simulink model "sma_simulator"  (R2019b)
settings: Solver=VariableStepAuto  StartTime=0.0  StopTime=200  FixedStep=0.01  MaxStep=0.01  RelTol=1e-3
PreLoadFcn:
  | load bus_type
model workspace (MAT data in the model file):
  Af = Simulink.Parameter
  Af.Value = 44.55
  Af.DataType = 'auto'
  Af.Dimensions = [1 1]
  As = Simulink.Parameter
  As.Value = 40.83
  As.DataType = 'auto'
  As.Dimensions = [1 1]
  C1 = Simulink.Parameter
  C1.Value = Simulink.data.Expression
  C1.Value.ExpressionString = " 8 * W_c * D_s / (pi * d_s^3)"
  C1.DataType = 'auto'
  C1.Dimensions = -1
  C2 = Simulink.Parameter
  C2.Value = Simulink.data.Expression
  C2.Value.ExpressionString = " d_s / (pi * N * D_s^2)"
  C2.DataType = 'auto'
  C2.Dimensions = -1
  C_A = Simulink.Parameter
  C_A.Value = 39.55
  C_A.DataType = 'auto'
  C_A.Dimensions = [1 1]
  C_M = Simulink.Parameter
  C_M.Value = 11.51
  C_M.DataType = 'auto'
  C_M.Dimensions = [1 1]
  D_s = Simulink.Parameter
  D_s.Value = Simulink.data.Expression
  D_s.Value.ExpressionString = "d_s+4.75e-3"
  D_s.DataType = 'auto'
  D_s.Dimensions = -1
  G_A = Simulink.Parameter
  G_A.Value = 18750000000
  G_A.DataType = 'auto'
  G_A.Dimensions = [1 1]
  G_M = Simulink.Parameter
  G_M.Value = 14390000000
  G_M.DataType = 'auto'
  G_M.Dimensions = [1 1]
  Mf = Simulink.Parameter
  Mf.Value = 26.41
  Mf.DataType = 'auto'
  Mf.Dimensions = [1 1]
  Ms = Simulink.Parameter
  Ms.Value = 29.74
  Ms.DataType = 'auto'
  Ms.Dimensions = [1 1]
  N = Simulink.Parameter
  N.Value = 25
  N.DataType = 'auto'
  N.Dimensions = [1 1]
  R = Simulink.Parameter
  R.Value = Simulink.data.Expression
  R.Value.ExpressionString = "D_s/d_s"
  R.DataType = 'auto'
  R.Dimensions = -1
  Sig = Simulink.Signal
  Sig.DataType = 'auto'
  Sig.Dimensions = -1
  Sig.DimensionsMode = 'auto'
  Sig.Complexity = 'auto'
  Sig.SampleTime = -1
  Sig.SamplingMode = 'auto'
  W_c = Simulink.Parameter
  W_c.Value = Simulink.data.Expression
  W_c.Value.ExpressionString = "(4*R-1)/(4*R-4)+0.615/R"
  W_c.DataType = 'auto'
  W_c.Dimensions = -1
  a_A = Simulink.Parameter
  a_A.Value = Simulink.data.Expression
  a_A.Value.ExpressionString = "pi/(Af - As)"
  a_A.DataType = 'auto'
  a_A.Dimensions = -1
  a_M = Simulink.Parameter
  a_M.Value = Simulink.data.Expression
  a_M.Value.ExpressionString = "pi/(Ms - Mf)"
  a_M.DataType = 'auto'
  a_M.Dimensions = -1
  d_s = Simulink.Parameter
  d_s.Value = 0.0015
  d_s.DataType = 'auto'
  d_s.Dimensions = [1 1]
  gamma_L = Simulink.Parameter
  gamma_L.Value = 0.02
  gamma_L.DataType = 'auto'
  gamma_L.Dimensions = [1 1]
  tau_fcr = Simulink.Parameter
  tau_fcr.Value = 320000000
  tau_fcr.DataType = 'auto'
  tau_fcr.Dimensions = [1 1]
  tau_scr = Simulink.Parameter
  tau_scr.Value = 60000000
  tau_scr.DataType = 'auto'
  tau_scr.Dimensions = [1 1]
undefined symbols (not defined in the file or in its folder): sigbuilder_block
libraries: simulink x3
Description:
  | -> System Requirement <-
  | - Matlab 2019b
  | - Simulink with licence to
  |   - Stateflow
settings Model: PauseTimes=128  OrderedModelArguments=off  Creator=Quinn Ding  LastModifiedBy=Quinn

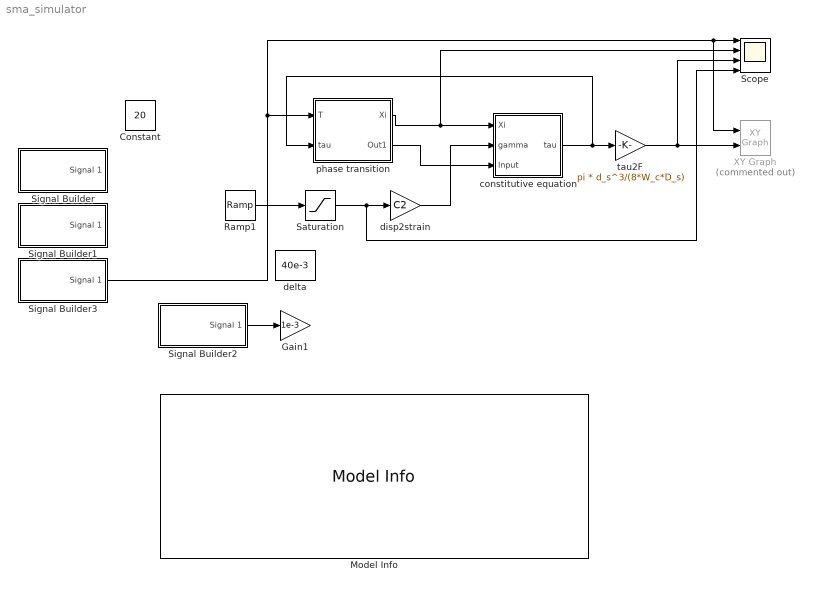
== system sma_simulator ==
  Constant : Constant  Value=20
  Gain1 : Gain  Gain=1e-3
  Model Info : simulink/Model-Wide Utilities/Model Info  Frame=on  DisplayStringWithTags=|  HorizontalTextAlignment=Left  LeftAlignmentValue=0.02
      | Shape Memory Alloy Simulator %<ModelVersion>
      | 
      | Developed by %<Creator> at Surgical Robotics & Devices Laboratory, CUHK.
      | 
      | %<Description>
      | 
      | Last modified on %<LastModificationDate>
  Ramp1 : simulink/Sources/Ramp  slope=1e-3  start=0  InitialOutput=0
  Saturation : Saturate  UpperLimit=40e-3  LowerLimit=0
  Scope : Scope  NumInputPorts=4
  Signal Builder : Subsystem  Tag=STV Subsys  LoadFcn=sigbuilder_block('load');  StartFcn=sigbuilder_block('start');  StopFcn=sigbuilder_block('stop');  ClipboardFcn=sigbuilder_block('clipboard');  mask(Sigbuilder block){tuvar=[0:10]}
      mask help: Simulink:masks:SigbuilderBlock_MD
      mask init:
      | if ~strcmp(get_param(bdroot(gcbh),'SimulationStatus'),'stopped') tuvar = sigbuilder_block('maskInit'); end
      settings: CopyFcn=sigbuilder_block('copy');  DeleteFcn=sigbuilder_block('delete');  ModelCloseFcn=sigbuilder_block('modelClose');  PreSaveFcn=sigbuilder_block('preSave');  PauseFcn=sigbuilder_block('pause');  ContinueFcn=sigbuilder_block('continue');  NameChangeFcn=sigbuilder_block('namechange');  OpenFcn=sigbuilder_block('open',[6 44.25 1428 681.75 ]);  CloseFcn=sigbuilder_block('close');
      mask Display: plot(0, 0, 100, 100,[2, 2, 32, 32, 2], [68, 8, 8, 68, 68],[32, 2], [38, 38], [32, 19, 2],[53, 60, 44], [32, 17, 17, 2],[16, 16, 31, 31]);txt = getActiveGroup(gcbh);text(2, 100, txt,'verticalAlignment', 'top');
  Signal Builder1 : Subsystem  Tag=STV Subsys  LoadFcn=sigbuilder_block('load');  StartFcn=sigbuilder_block('start');  StopFcn=sigbuilder_block('stop');  ClipboardFcn=sigbuilder_block('clipboard');  mask(Sigbuilder block){tuvar=[0:10]}
      mask help: Simulink:masks:SigbuilderBlock_MD
      mask init:
      | if ~strcmp(get_param(bdroot(gcbh),'SimulationStatus'),'stopped') tuvar = sigbuilder_block('maskInit'); end
      settings: CopyFcn=sigbuilder_block('copy');  DeleteFcn=sigbuilder_block('delete');  ModelCloseFcn=sigbuilder_block('modelClose');  PreSaveFcn=sigbuilder_block('preSave');  PauseFcn=sigbuilder_block('pause');  ContinueFcn=sigbuilder_block('continue');  NameChangeFcn=sigbuilder_block('namechange');  OpenFcn=sigbuilder_block('open',[6 44.25 1428 681.75 ]);  CloseFcn=sigbuilder_block('close');
      mask Display: plot(0, 0, 100, 100,[2, 2, 32, 32, 2], [68, 8, 8, 68, 68],[32, 2], [38, 38], [32, 19, 2],[53, 60, 44], [32, 17, 17, 2],[16, 16, 31, 31]);txt = getActiveGroup(gcbh);text(2, 100, txt,'verticalAlignment', 'top');
  Signal Builder2 : Subsystem  Tag=STV Subsys  LoadFcn=sigbuilder_block('load');  StartFcn=sigbuilder_block('start');  StopFcn=sigbuilder_block('stop');  ClipboardFcn=sigbuilder_block('clipboard');  mask(Sigbuilder block){tuvar=[0:10]}
      mask help: Simulink:masks:SigbuilderBlock_MD
      mask init:
      | if ~strcmp(get_param(bdroot(gcbh),'SimulationStatus'),'stopped') tuvar = sigbuilder_block('maskInit'); end
      settings: CopyFcn=sigbuilder_block('copy');  DeleteFcn=sigbuilder_block('delete');  ModelCloseFcn=sigbuilder_block('modelClose');  PreSaveFcn=sigbuilder_block('preSave');  PauseFcn=sigbuilder_block('pause');  ContinueFcn=sigbuilder_block('continue');  NameChangeFcn=sigbuilder_block('namechange');  OpenFcn=sigbuilder_block('open',[6 44.25 1428 681.75 ]);  CloseFcn=sigbuilder_block('close');
      mask Display: plot(0, 0, 100, 100,[2, 2, 32, 32, 2], [68, 8, 8, 68, 68],[32, 2], [38, 38], [32, 19, 2],[53, 60, 44], [32, 17, 17, 2],[16, 16, 31, 31]);txt = getActiveGroup(gcbh);text(2, 100, txt,'verticalAlignment', 'top');
  Signal Builder3 : Subsystem  Tag=STV Subsys  LoadFcn=sigbuilder_block('load');  StartFcn=sigbuilder_block('start');  StopFcn=sigbuilder_block('stop');  ClipboardFcn=sigbuilder_block('clipboard');  mask(Sigbuilder block){tuvar=[0:10]}
      mask help: Simulink:masks:SigbuilderBlock_MD
      mask init:
      | if ~strcmp(get_param(bdroot(gcbh),'SimulationStatus'),'stopped') tuvar = sigbuilder_block('maskInit'); end
      settings: CopyFcn=sigbuilder_block('copy');  DeleteFcn=sigbuilder_block('delete');  ModelCloseFcn=sigbuilder_block('modelClose');  PreSaveFcn=sigbuilder_block('preSave');  PauseFcn=sigbuilder_block('pause');  ContinueFcn=sigbuilder_block('continue');  NameChangeFcn=sigbuilder_block('namechange');  OpenFcn=sigbuilder_block('open',[6 44.25 1155 593.25 ]);  CloseFcn=sigbuilder_block('close');
      mask Display: plot(0, 0, 100, 100,[2, 2, 32, 32, 2], [68, 8, 8, 68, 68],[32, 2], [38, 38], [32, 19, 2],[53, 60, 44], [32, 17, 17, 2],[16, 16, 31, 31]);txt = getActiveGroup(gcbh);text(2, 100, txt,'verticalAlignment', 'top');
  XY Graph : simulink/Sinks/XY Graph  Commented=on  xmin=20  xmax=80  ymin=0  ymax=100  st=-1
  constitutive equation : Subsystem
  delta : Constant  Value=40e-3
  disp2strain : Gain  Gain=C2
  phase transition : Subsystem
  tau2F : Gain  Gain=pi * d_s^3/(8*W_c*D_s)
  wires:
  Signal Builder3/1(Signal 1) -> XY Graph/1, Scope/1, phase transition/1(T)
  constitutive equation/1(tau) -> phase transition/2(tau), tau2F/1
  phase transition/1(Xi) -> constitutive equation/1(Xi), Scope/2
  tau2F/1 -> XY Graph/2, Scope/3
  Ramp1/1 -> Saturation/1
  disp2strain/1 -> constitutive equation/2(gamma)
  Signal Builder2/1(Signal 1) -> Gain1/1
  Saturation/1 -> Scope/4, disp2strain/1
  phase transition/2(Out1) -> constitutive equation/3(Input)

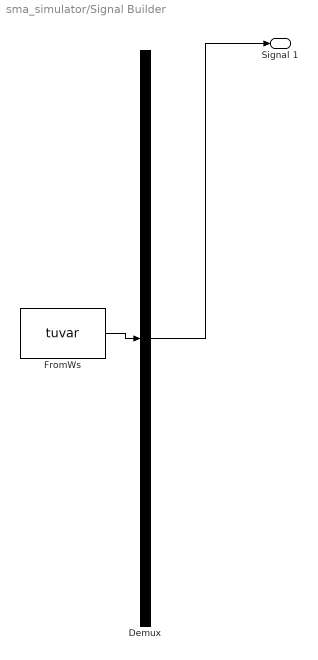
== system sma_simulator/Signal Builder ==
  Demux : Demux  Tag=STV Demux  Outputs=1
  FromWs : FromWorkspace  Tag=STV FromWs  VariableName=tuvar  SampleTime=0
      SigBuilderData=|
      | common.afterFinalStr = 'Extrapolate'
      | common.sampleTime = 0
      | dataSet.timeRange = [0 80]
      | dataSet.name = 'Group 1'
      | sbobj.Groups.Name = 'Group 1'
      | sbobj.Groups.Signals.Name = 'Signal 1'
      | sbobj.Groups.Signals.XData = [0 5 10 15 20 25 30 35 40 45 50 55 60 65 70 75 80]
      | sbobj.Groups.Signals.YData = [20 20 60 60 20 42 42 20 20 42 42 28 28 60 60 28 28]
      | sbobj.Groups.TimeRange = [0 80]
  Signal 1 : Outport  Tag=STV Outport
  wires:
  Demux/1 -> Signal 1/1
  FromWs/1 -> Demux/1

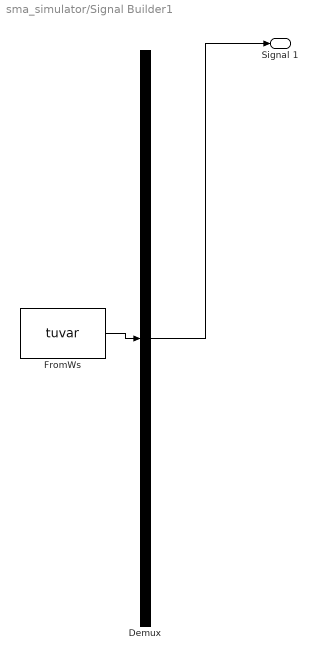
== system sma_simulator/Signal Builder1 ==
  Demux : Demux  Tag=STV Demux  Outputs=1
  FromWs : FromWorkspace  Tag=STV FromWs  VariableName=tuvar  SampleTime=0
      SigBuilderData=|
      | common.afterFinalStr = 'Extrapolate'
      | common.sampleTime = 0
      | dataSet.timeRange = [0 80]
      | dataSet.name = 'Group 1'
      | sbobj.Groups.Name = 'Group 1'
      | sbobj.Groups.Signals.Name = 'Signal 1'
      | sbobj.Groups.Signals.XData = [0 5 35 45 75 80]
      | sbobj.Groups.Signals.YData = [20 20 60 60 20 20]
      | sbobj.Groups.TimeRange = [0 80]
  Signal 1 : Outport  Tag=STV Outport
  wires:
  Demux/1 -> Signal 1/1
  FromWs/1 -> Demux/1

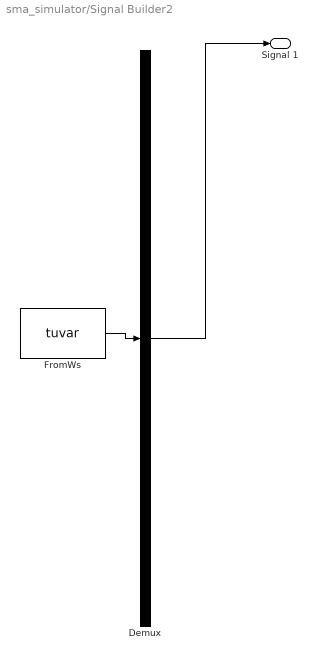
== system sma_simulator/Signal Builder2 ==
  Demux : Demux  Tag=STV Demux  Outputs=1
  FromWs : FromWorkspace  Tag=STV FromWs  VariableName=tuvar  SampleTime=0
      SigBuilderData=|
      | common.afterFinalStr = 'Extrapolate'
      | common.sampleTime = 0
      | dataSet.timeRange = [0 80]
      | dataSet.name = 'Group 1'
      | sbobj.Groups.Name = 'Group 1'
      | sbobj.Groups.Signals.Name = 'Signal 1'
      | sbobj.Groups.Signals.XData = [0 5 35 45 75 80]
      | sbobj.Groups.Signals.YData = [0 0 150 150 0 0]
      | sbobj.Groups.TimeRange = [0 80]
  Signal 1 : Outport  Tag=STV Outport
  wires:
  Demux/1 -> Signal 1/1
  FromWs/1 -> Demux/1

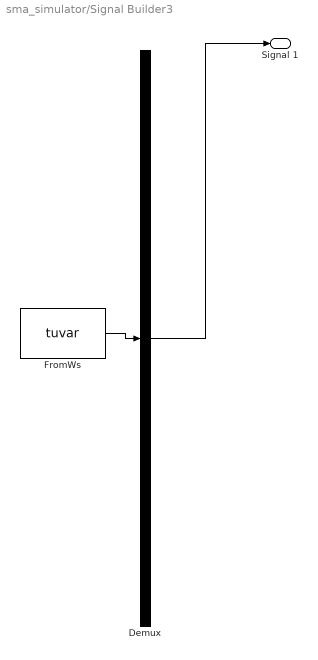
== system sma_simulator/Signal Builder3 ==
  Demux : Demux  Tag=STV Demux  Outputs=1
  FromWs : FromWorkspace  Tag=STV FromWs  VariableName=tuvar  SampleTime=0
      SigBuilderData=|
      | common.afterFinalStr = 'Extrapolate'
      | common.sampleTime = 0
      | dataSet.timeRange = [0 200]
      | dataSet.name = 'Group 1'
      | sbobj.Groups.Name = 'Group 1'
      | sbobj.Groups.Signals.Name = 'Signal 1'
      | sbobj.Groups.Signals.XData = [0 110 140 150 180 200]
      | sbobj.Groups.Signals.YData = [20 20 60 60 20 20]
      | sbobj.Groups.TimeRange = [0 200]
  Signal 1 : Outport  Tag=STV Outport
  wires:
  FromWs/1 -> Demux/1
  Demux/1 -> Signal 1/1

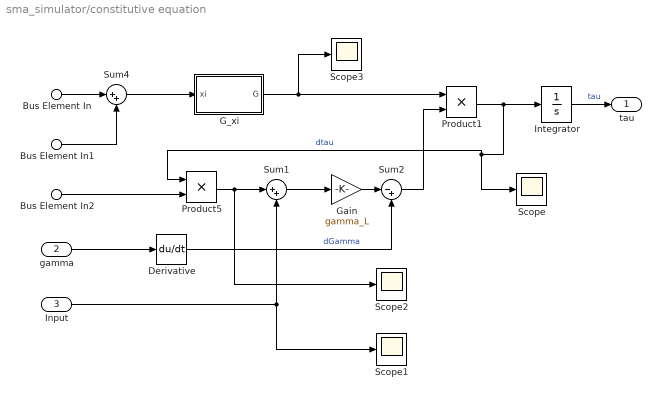
== system sma_simulator/constitutive equation ==
  Bus Element In : Inport  PortName=Xi  Element=xi_S
  Bus Element In1 : Inport  PortName=Xi  Element=xi_T
  Bus Element In2 : Inport  PortName=Xi  Element=dxi_S
  gamma : Inport  Port=2
  Input : Inport  Port=3
  Derivative : Derivative
  G_xi : Subsystem
  Gain : Gain  Gain=gamma_L
  Integrator : Integrator
  Product1 : Product
  Product5 : Product
  Scope{,1..3} (4 alike) : Scope
  Sum1 : Sum  Inputs=|++
  Sum2 : Sum  Inputs=|-+
  Sum4 : Sum  Inputs=|++
  tau : Outport
  wires:
  Bus Element In/1 -> Sum4/1
  Bus Element In1/1 -> Sum4/2
  G_xi/1(G) -> Scope3/1, Product1/1
  Derivative/1 -> Sum2/2  "dGamma"
  Gain/1 -> Sum2/1
  gamma/1 -> Derivative/1
  Sum2/1 -> Product1/2
  Product1/1 -> Scope/1, Product5/1, Integrator/1  "dtau"
  Bus Element In2/1 -> Product5/2
  Integrator/1 -> tau/1  "tau"
  Sum1/1 -> Gain/1
  Sum4/1 -> G_xi/1(xi)
  Product5/1 -> Scope2/1, Sum1/1
  Input/1 -> Scope1/1, Sum1/2

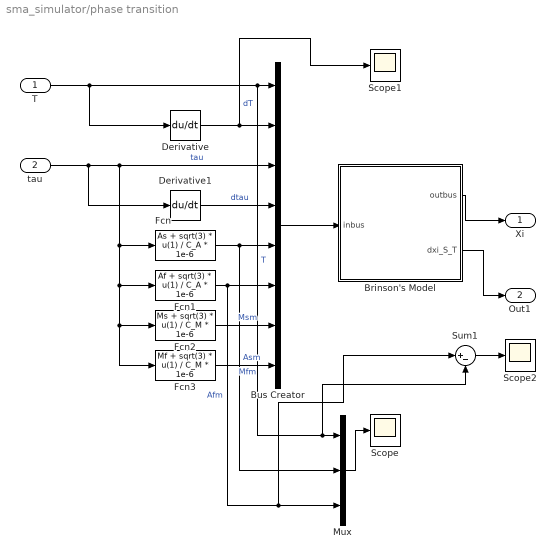
== system sma_simulator/phase transition ==
  T : Inport
  tau : Inport  Port=2
  Brinson's Model : Stateflow chart  BlockKeywords=__PRM__SERIALIZED__DATA__:Stateflow Chart,Stateflow Diagram  TreatAsAtomicUnit=on
  Bus Creator : BusCreator  Inputs=8  OutDataTypeStr=Bus: phase_tran_in_bus
  Derivative : Derivative
  Derivative1 : Derivative
  Fcn : Fcn  Expr=As + sqrt(3) * u(1) / C_A * 1e-6
  Fcn1 : Fcn  Expr=Af + sqrt(3) * u(1) / C_A * 1e-6
  Fcn2 : Fcn  Expr=Ms + sqrt(3) * u(1) / C_M * 1e-6
  Fcn3 : Fcn  Expr=Mf + sqrt(3) * u(1) / C_M * 1e-6
  Mux : Mux  Inputs=3
  Scope : Scope
  Scope1 : Scope
  Scope2 : Scope
  Sum1 : Sum  Inputs=|+-
  Xi : Outport  OutDataTypeStr=Bus: phase_tran_out_bus
  Out1 : Outport  Port=2
  wires:
  tau/1 -> Bus Creator/3, Fcn/1, Fcn1/1, Fcn2/1, Fcn3/1, Derivative1/1  "tau"
  Fcn1/1 -> Sum1/1, Mux/3, Bus Creator/6  "Afm"
  Bus Creator/1 -> Brinson's Model/1(inbus)
  Derivative1/1 -> Bus Creator/4  "dtau"
  Fcn2/1 -> Bus Creator/7  "Msm"
  Derivative/1 -> Scope1/1, Bus Creator/2  "dT"
  Fcn/1 -> Mux/2, Bus Creator/5  "Asm"
  T/1 -> Sum1/2, Mux/1, Bus Creator/1, Derivative/1  "T"
  Fcn3/1 -> Bus Creator/8  "Mfm"
  Brinson's Model/1(outbus) -> Xi/1
  Brinson's Model/2(dxi_S_T) -> Out1/1
  Mux/1 -> Scope/1
  Sum1/1 -> Scope2/1

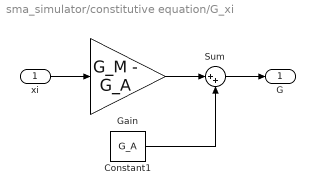
== system sma_simulator/constitutive equation/G_xi ==
  xi : Inport
  Constant1 : Constant  Value=G_A
  Gain : Gain  Gain=G_M - G_A
  Sum : Sum  Inputs=|++
  G : Outport
  wires:
  Constant1/1 -> Sum/2
  Gain/1 -> Sum/1
  Sum/1 -> G/1
  xi/1 -> Gain/1

== stateflow chart sma_simulator/phase transition/Brinson's Model ==
  state Austenite
    entry:
    xi = 0;
  state MixedState
    state A2M
      entry:
      xi_0 = xi;
      during:
      xi = (1 - xi_0) / 2 * cos(a_M * (inbus.T - inbus.Mfm)) + (1 + xi_0) / 2;
    state DeadZone
    state M2A
      entry:
      xi_0 = xi;
      during:
      xi = xi_0 / 2 * (cos(a_A * (inbus.T - inbus.Asm)) + 1);
    (default) -> A2M
    A2M -> DeadZone : [inbus.dT > 0]
    DeadZone -> A2M [order 1] : [inbus.dT < 0 && inbus.T < inbus.Msm]
    MixedState.M2A -> DeadZone : [inbus.dT < 0]
    DeadZone -> MixedState.M2A [order 2] : [inbus.dT > 0 && inbus.T > inbus.Asm]
  state TIM2
    entry:
    outbus.xi_S = 0;
    outbus.xi_T = 1;
  state Martensite
    state PureStressInduced
      en:
      xi_S0 = outbus.xi_S;
      xi_T0 = outbus.xi_T;
      du:
      outbus.xi_S = (1 - xi_S0) / 2 * cos(pi / (tau_scr - tau_fcr) * (inbus.tau - tau_fcr - C_M * (inbus.T - Ms))) + (1 + xi_S0) / 2;
      outbus.xi_T = xi_T0 - xi_T0 / (1 - xi_S0) * (outbus.xi_S - xi_S0);
    state FullSIM
      en:
      outbus.xi_S = 1;
      outbus.xi_T = 0;
    state FullTIM
      en:
      outbus.xi_S = 0;
      outbus.xi_T = 1;
    state MixedM1
      en:
      xi_S0 = outbus.xi_S;
      xi_T0 = outbus.xi_T;
      du:
      outbus.xi_S = (1 - xi_S0) / 2 * cos(pi / (tau_scr - tau_fcr) * (inbus.tau - tau_fcr)) + (1 + xi_S0) / 2;
      outbus.xi_T = xi_T0 - xi_T0 / (1 - xi_S0) * (outbus.xi_S - xi_S0);
      state NoTIM
      state TIM
      (default) -> NoTIM
    (default) -> FullTIM
    PureStressInduced -> FullSIM : [outbus.xi_S >= 1]
    FullTIM -> PureStressInduced [order 1] : [inbus.T > Ms && (tau_scr + C_M * (inbus.T - Ms)) < inbus.tau && inbus.tau < (tau_fcr + C_M * (inbus.T - Ms))]
    FullTIM -> MixedM1 [order 2] : [inbus.T < Ms && tau_scr < inbus.tau && inbus.tau < tau_fcr]
  state A
    en:
    outbus.xi_S = 0;
    outbus.xi_T = 0;
    outbus.dxi_S = 0;
    dxi_S_T = 0；
  state Hysteresis
    en:
    outbus.dxi_S = 0;
  state o
    en:
    xi_S0 = outbus.xi_S;
    xi_T0 = outbus.xi_T;
    du:
    outbus.xi_S = ...
    (1 - xi_S0) / 2 * cos(pi / (tau_scr - tau_fcr) * (inbus.tau - tau_fcr)) + ...
    (1 + xi_S0) / 2;
    outbus.xi_T = ...
    xi_T0 - xi_T0 / (1 - xi_S0) * (outbus.xi_S - xi_S0);
    outbus.dxi_S = ....
    -(1 - xi_S0) / 2 * sin(pi / (tau_scr - tau_fcr) * (inbus.tau - tau_fcr)) * ...
    pi / (tau_scr - tau_fcr);
    dxi_S_T = 0；
  state M_ot
    en:
    xi = 1;
    xi_0 = 1;
  state M2A
    en:
    xi_0 = outbus.xi_S + outbus.xi_T;
    xi_S0 = outbus.xi_S;
    xi_T0 = outbus.xi_T;
    du:
    xi = ...
    xi_0 / 2 * (cos(a_A * (inbus.T - inbus.Asm)) + 1);
    outbus.xi_S = xi_S0 - xi_S0 / xi_0 * (xi_0 - xi);
    outbus.xi_T = xi_T0 - xi_T0 / xi_0 * (xi_0 - xi);
    outbus.dxi_S = ....
    xi_S0 / 2 * sin(a_A * (inbus.T - inbus.Asm)) * ...
    a_A  / C_A * 1e-6;
    dxi_S_T = ...
    -xi_S0 / 2 * sin(a_A * (inbus.T - inbus.Asm)) * ...
    a_A * inbus.dT;
  state M_o
    en:
    outbus.xi_S = 1;
    outbus.xi_T = 0;
    outbus.dxi_S = 0;
    dxi_S_T = 0；
  Austenite -> MixedState : [inbus.T < inbus.Msm]
  MixedState -> Austenite [order 2] : [inbus.T > inbus.Afm]
  TIM2 -> MixedState : [inbus.T > inbus.Asm]
  MixedState -> TIM2 [order 1] : [inbus.T < inbus.Mfm]
  M2A -> Hysteresis [order 2] : [inbus.dT < 0]
  (default) -> M_ot : {outbus = struct( ...
      | 'xi_S', {0}, ...
      | 'xi_T', {1}, ...
      | 'dxi_S', {0});}
  Hysteresis -> M2A [order 2] : [inbus.dT > 0]
  o -> Hysteresis [order 1] : [inbus.dtau < 0]
  Hysteresis -> o [order 1] : [inbus.dtau > 0]
  M2A -> A [order 1] : [inbus.T > inbus.Afm]
  M_ot -> o [order 1] : [inbus.T < Mf && ...
      | tau_scr < inbus.tau && ...
      | inbus.tau < tau_fcr]
  M_ot -> M2A [order 2] : [inbus.T > inbus.Asm]
  o -> M2A [order 3] : [inbus.T > inbus.Asm]
  o -> M_o [order 2] : [inbus.tau > tau_fcr]
  M_o -> M2A : [inbus.T > inbus.Asm]
  data: xi_0 local; a_M parameter; a_A parameter; inbus input Bus: phase_tran_in_bus; xi_S0 local; xi_T0 local; C_M parameter; Ms parameter; tau_scr parameter; tau_fcr parameter; Mf parameter; outbus output Bus: phase_tran_out_bus; xi local; C_A parameter; dxi_S_T output
